simulink library "dch"  (Simulink 8.1)
settings: Solver=ode1  StartTime=0.0  StopTime=Inf  FixedStep=0.001  RelTol=1e-3
PostLoadFcn:
  | , if any(exist('dsrtsu_mdlpostloadfcn', 'file') == [2, 3, 6]), try dsrtsu_mdlpostloadfcn('Execute', bdroot); catch fprintf('Error in PostLoadFcn (dsrtsu_mdlpostloadfcn) for model "%s":\n %s\n', bdroot, lasterr); end, end,
undefined symbols (not defined in the file or in its folder): KACC_DistControlDisableSpd_kph, KACC_DistControlEnableSpd_kph
libraries: hcu_lib x3
settings Model: DSRTSU_INTERNAL_RTI_VER=450  DSRTSU_INTERNAL_RTI_TYPE=rti1401  RTICANMMDATA=struct('GeneralSetupData',struct('modelroot','D:\ELN150201_TAIWAN\trunk\AdasDragon\software\sw_development\arch\app\acc','generalsettings',struct('filesettings',struct('destfolder',struct('Name','RTICANMM_FILES','Check',1),'buildfolder',struct('Name','.','Check',1),'AbsDestfolder',struct('Name','D:\ELN150201_TAIWAN\trunk\AdasDragon\software\sw_development\arch\app\acc\RTICANMM_FILES'),'AbsBuildfolder',struct('Name','D:\ELN150201_TAIWAN\trunk\AdasDragon\software\sw_development\arch\app\acc'))),'options',struct('addpaths',1,'rmpaths',1,'addtrcexclusion',logical(1),'cannavigator',struct('checkmonitoring',0),'show_usrtrc',0,'use_usrtrc',0),'advanced',struct('options',[1 1 1 1 1 1 1 1 1 1 1 1 1 1 1 1 1 1 1 1 1 1 1 1 1 1 1 1 1 1 1 1 1 1 1 1 1 1 1 1 1 1 1 1 1 1 1 1 1 1 1 1 1 1 1 1 1 1 1 1 1 1 1 1 1 1 1 1 1 1 1 1 1 1 1 1 1 1 1 1 1 1 1 1 1 1 1 1 1 1 1 1 1 1 1 1 1 1 1 1]),'MPSetup',{{}},'modelname','dch','block','dch'))  DSRTSU_INTERNAL_RTIFPGA=40  Creator=AT015411  LastModifiedBy=AT015555

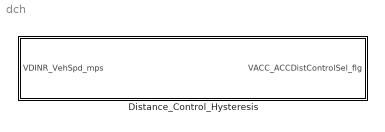
== system dch ==
  Distance_Control_Hysteresis : Subsystem

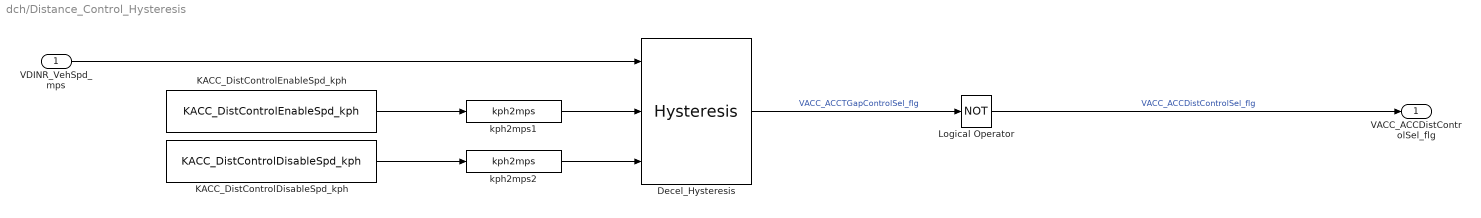
== system dch/Distance_Control_Hysteresis ==
  VDINR_VehSpd_mps : Inport
  Decel_Hysteresis : hcu_lib/Hysteresis  SystemSampleTime=-1
  KACC_DistControlDisableSpd_kph : Constant  Value=KACC_DistControlDisableSpd_kph
  KACC_DistControlEnableSpd_kph : Constant  Value=KACC_DistControlEnableSpd_kph
  Logical Operator : Logic  Operator=NOT  AllPortsSameDT=off  OutDataTypeStr=boolean
  kph2mps1 : hcu_lib/kph2mps
  kph2mps2 : hcu_lib/kph2mps
  VACC_ACCDistControlSel_flg : Outport
  wires:
  Decel_Hysteresis/1 -> Logical Operator/1  "VACC_ACCTGapControlSel_flg"
  kph2mps2/1 -> Decel_Hysteresis/3
  KACC_DistControlDisableSpd_kph/1 -> kph2mps2/1
  kph2mps1/1 -> Decel_Hysteresis/2
  Logical Operator/1 -> VACC_ACCDistControlSel_flg/1  "VACC_ACCDistControlSel_flg"
  VDINR_VehSpd_mps/1 -> Decel_Hysteresis/1
  KACC_DistControlEnableSpd_kph/1 -> kph2mps1/1
